simulink model "Demo_MinSegMotor_Nano33IoT_25a_PositionControl"  (R2025a)
settings: Solver=FixedStepDiscrete  StartTime=0.0  StopTime=inf  FixedStep=.005  RelTol=1e-3
libraries: arduinolib x2, arduinosensorlib x1
settings Model: SILPILModeSetting=veronly  ExtModeTrigDuration=2  Creator=Alec  LastModifiedBy=hurstj
settings SolverCC: AlgebraicLoopSolver=TrustRegion
settings DataIOCC: LimitDataPoints=on  SaveFormat=Array  SaveOutput=off  DSMLogging=off  SaveTime=off  ReturnWorkspaceOutputs=off
settings OptimizationCC: EnhancedBackFolding=on  PassReuseOutputArgsThreshold=0.0  ExpressionDepthLimit=2147483647.0  MaxStackSize=64  OptimizeBlockOrder=speed  DifferentSizesBufferReuse=on  OptimizationCustomize=off
settings DebuggingCC: UnderspecifiedInitializationDetection=Classic  MergeDetectMultiDrivingBlocksExec=none  ParameterTunabilityLossMsg=error  UnconnectedInputMsg=warning  UnconnectedOutputMsg=warning  UnconnectedLineMsg=warning  StateNameClashWarn=warning  SFUnexpectedBacktrackingDiag=warning  SFNoUnconditionalDefaultTransitionDiag=warning  SFExecutionAtInitializationDiag=none  ArithmeticOperatorsInVariantConditions=warning
settings HardwareCC: ProdBitPerPointer=32.0  ProdBitPerSizeT=32.0  ProdBitPerPtrDiffT=32.0  ProdLargestAtomicInteger=Long  ProdLargestAtomicFloat=Double  ProdWordSize=32.0  ProdHWDeviceType=ARM Compatible->ARM Cortex  UseEmbeddedCoderFeatures=off  UseSimulinkCoderFeatures=off
settings ModelReferenceCC: EnableRefExpFcnMdlSchedulingChecks=on  PropagateSignalLabelsOutOfModel=off
settings SFSimCC: SimUseLocalCustomCode=off  MATLABDynamicMemAlloc=off  CustomCodeUndefinedFunction=UseInterfaceOnly
settings RTWCC: SystemTargetFile=ert.tlc  HardwareBoard=Arduino Nano 33 IoT  TemplateMakefile=ert_default_tmf  RTWVerbose=off  RTWUseLocalCustomCode=off  Toolchain=Arduino ARM  BuildConfiguration=Faster Runs  GPUComputeCapability=3.5  DLArmComputeVersion=19.05  Description=Embedded Coder
settings CodeAppCC: ForceParamTrailComments=on  OperatorAnnotations=on  MangleLength=10.0
settings ERTTargetCC: ExtModeTransport=3.0  ExtModeAutomaticAllocSize=off  ExtModeStaticAllocSize=8192.0  InlinedParameterPlacement=Hierarchical  DynamicArrayContainerType=coder::array  ERTCustomFileBanners=off  SupportContinuousTime=on  SupportNonInlinedSFcns=on  RemoveResetFunc=off  SupportVariableSizeSignals=on  ModelStepFunctionPrototypeControlCompliant=off
settings ConfigComp: CovMetricSettings=dw  CovSaveCumulativeToWorkspaceVar=on  CovSaveSingleToWorkspaceVar=on  CovExternalEMLEnable=off

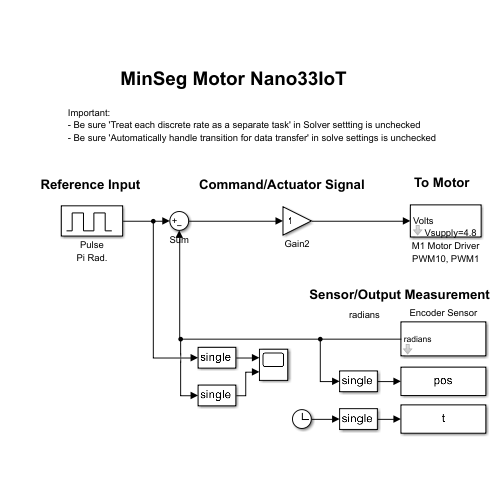
[thumbnail: Simulink's stored preview of the top-level diagram]
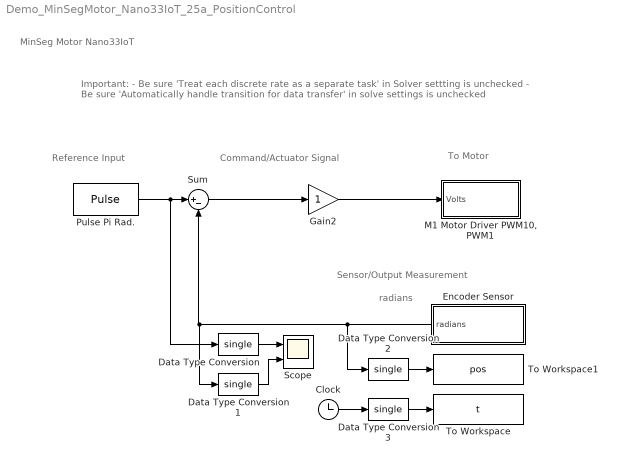
== system Demo_MinSegMotor_Nano33IoT_25a_PositionControl ==
  note: MinSeg Motor Nano33IoT
  note: Important:
      | - Be sure 'Treat each discrete rate as a separate task' in Solver settting is unchecked
      | - Be sure 'Automatically handle transition for data transfer' in solve settings is unchecked
  note: Reference Input
  note: Command/Actuator Signal
  note: To Motor
  note: Sensor/Output Measurement
  note: radians
  Clock : Clock
  Data Type Conversion{,1..3} (4 alike) : DataTypeConversion  OutDataTypeStr=single  SaturateOnIntegerOverflow=off  RndMeth=Floor
  Encoder Sensor : Subsystem
      mask DialogControl Control2 Prompt: Encoder Counter - unknown units
  Gain2 : Gain
  "M1 Motor Driver PWM10, PWM1" : Subsystem  mask{Vsupply=4.8, Voffset=0}
      mask prompts: Vsupply "Driver Voltage"
      mask help:
      | Specify driver supply voltage (around 4.9 for USB, 8.7 for 6AA batteries)
      | Specify the Voltage offset (0-Vsupply)
      |
      | Driver supply voltage can be measured direcly by turning the motor fully on (100% duty cycle) and measuring the voltage across the motor leads.  This is the maximum voltage available to the motor and is used to scale from volts to PWM value 0-255.
      |
      | Note this value must be changed if the supply voltage to the driver is changed, for example, by using batteries.
      |
      | Vsupply is the maximum voltage your system is capable of supplying to system given the power supply. It needs to be measured depending on the power supply.
      mask Display:
      | port_label('input',1,'Volts')
      | text(15,5,['Vsupply=' num2str(Vsupply)])
  Pulse Pi Rad. : DiscretePulseGenerator  PulseType=Time based  Amplitude=pi  Period=4  PulseWidth=50
  Scope : Scope  NumInputPorts=2
      settings: ActiveDisplayYMinimum=-1.4073676670460262  ActiveDisplayYMaximum=4.5301483885783957  DataLoggingVariableName=ScopeData3
  Sum : Sum  Inputs=|+-
  To Workspace : ToWorkspace  VariableName=t  SampleTime=-1
      settings: Save2DSignal=2-D array (concatenate along first dimension)
  To Workspace1 : ToWorkspace  VariableName=pos  SampleTime=-1
      settings: Save2DSignal=2-D array (concatenate along first dimension)
  wires:
  Clock/1 -> Data Type Conversion3/1
  Encoder Sensor/1(radians) -> Data Type Conversion2/1, Data Type Conversion1/1, Sum/2
  Sum/1 -> Gain2/1
  Pulse Pi Rad./1 -> Data Type Conversion/1, Sum/1
  Gain2/1 -> "M1 Motor Driver PWM10, PWM1"/1(Volts)
  Data Type Conversion/1 -> Scope/1
  Data Type Conversion1/1 -> Scope/2
  Data Type Conversion2/1 -> To Workspace1/1
  Data Type Conversion3/1 -> To Workspace/1

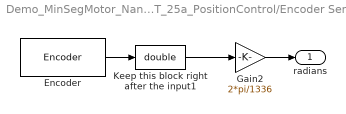
== system Demo_MinSegMotor_Nano33IoT_25a_PositionControl/Encoder Sensor ==
  Encoder : arduinosensorlib/Encoder  InputA=2  InputB=3  Mode=No reset  SampleTime=-1
  Gain2 : Gain  Gain=2*pi/1336
  Keep this block right after the input1 : DataTypeConversion  OutDataTypeStr=double  SaturateOnIntegerOverflow=off  RndMeth=Floor
  radians : Outport
  wires:
  Keep this block right after the input1/1 -> Gain2/1
  Gain2/1 -> radians/1
  Encoder/1 -> Keep this block right after the input1/1

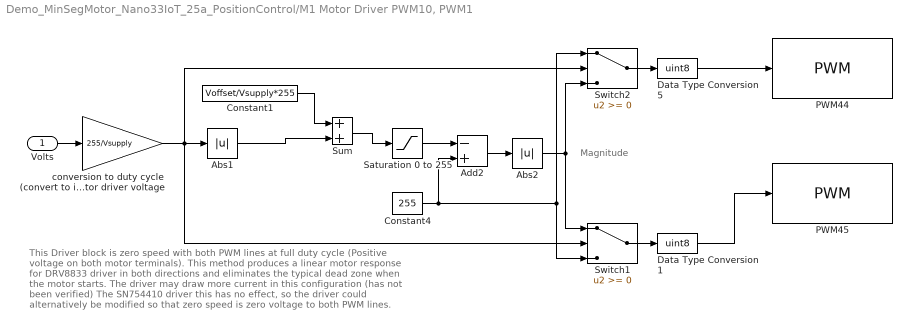
== system Demo_MinSegMotor_Nano33IoT_25a_PositionControl/M1 Motor Driver PWM10, PWM1 ==
  note: This Driver block is zero speed with both PWM lines at full duty cycle
      |  (Positive voltage on both motor terminals).
      | This method produces a linear motor response for DRV8833 driver
      |  in both directions and eliminates
      | the typical dead zone when the motor starts.
      | The driver may draw more current in this configuration (has not been verified)
      |
      | The SN754410 driver this has no effect, so the driver could alternatively
      | be modified so that zero speed is zero voltage to both PWM lines.
  note: Magnitude
  Volts : Inport
  Abs1 : Abs  SaturateOnIntegerOverflow=off
  Abs2 : Abs  SaturateOnIntegerOverflow=off
  Add2 : Sum  Inputs=-+
  Constant1 : Constant  Value=Voffset/Vsupply*255
  Constant4 : Constant  Value=255
  Data Type Conversion1 : DataTypeConversion  OutDataTypeStr=uint8  SaturateOnIntegerOverflow=off  RndMeth=Floor
  Data Type Conversion5 : DataTypeConversion  OutDataTypeStr=uint8  SaturateOnIntegerOverflow=off  RndMeth=Floor
  PWM44 : arduinolib/PWM  pinNumber=10  frequencyType=Specify  desiredFrequency=4000  achievableFrequency=4000
  PWM45 : arduinolib/PWM  pinNumber=12  frequencyType=Specify  desiredFrequency=4000  achievableFrequency=3989.3617
  Saturation 0 to 255 : Saturate  UpperLimit=255  LowerLimit=0
  Sum : Sum
  Switch1 : Switch  SaturateOnIntegerOverflow=off  InputSameDT=off
  Switch2 : Switch  SaturateOnIntegerOverflow=off  InputSameDT=off
  conversion to duty cycle (convert to int) denominator is motor driver voltage : Gain  Gain=255/Vsupply  OutDataTypeStr=int16
  wires:
  Abs1/1 -> Sum/2
  Sum/1 -> Saturation 0 to 255/1
  Constant1/1 -> Sum/1
  Volts/1 -> conversion to duty cycle (convert to int) denominator is motor driver voltage/1
  conversion to duty cycle (convert to int) denominator is motor driver voltage/1 -> Switch2/2, Abs1/1, Switch1/2
  Saturation 0 to 255/1 -> Add2/1
  Constant4/1 -> Switch1/3, Switch2/1, Add2/2
  Add2/1 -> Abs2/1
  Abs2/1 -> Switch2/3, Switch1/1
  Switch2/1 -> Data Type Conversion5/1
  Switch1/1 -> Data Type Conversion1/1
  Data Type Conversion5/1 -> PWM44/1
  Data Type Conversion1/1 -> PWM45/1
